simulink model "bolide"  (R2025a)
settings: Solver=VariableStepAuto  StartTime=0.0  StopTime=10.0  RelTol=1e-3
InitFcn:
  | run("init.m")
model workspace (MATLAB code in the model file):
  | % Définition des constantes
  | 
  | rho = 0.04; % rayon des roues
  | k = 0.0854; % constante de couple
  | R = 3.87; % résistance des moteurs
  | d = 0.05; % distance entre le centre des roues et le centre de masse
  | l = 0.16; % distance entre les roues
  | mb = 2; % masse du châssis du robot
  | mw = 0.5; % masse d'une unité
  | M = 2*mw + mb; % masse du robot
  | Ix = 8.48e-3; % moments d'inertie du robot
  | Iz = 1.233e-2;
  | Ixw  = 4.00e-4;    % roue - inertie de rotation autour de l'axe (spin)
  | Izw  = 4.00e-4;    % roue - inertie (même ordre que Ixw)
  | Iyw  = 2.375e-4;   % roue - inertie transversale (axe perpendiculaire au spin)
  | Ipsi = Ix + Iz + Ixw + Izw + mw*(l^2)/2 + Iyw*(l^2)/(2*(rho^2));
  | A = M + 2*Iyw*(rho^2);
  | B = Ipsi + mb*(d^2);
  | D = A*B + 2*(mb*d/2)^2;
settings Model: Creator=arthu  LastModifiedBy=arthu

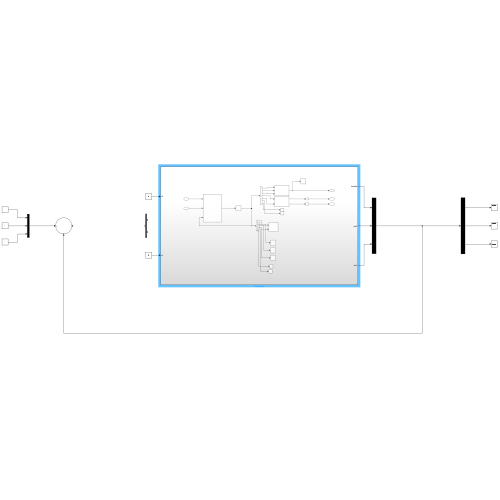
[thumbnail: Simulink's stored preview of the top-level diagram]
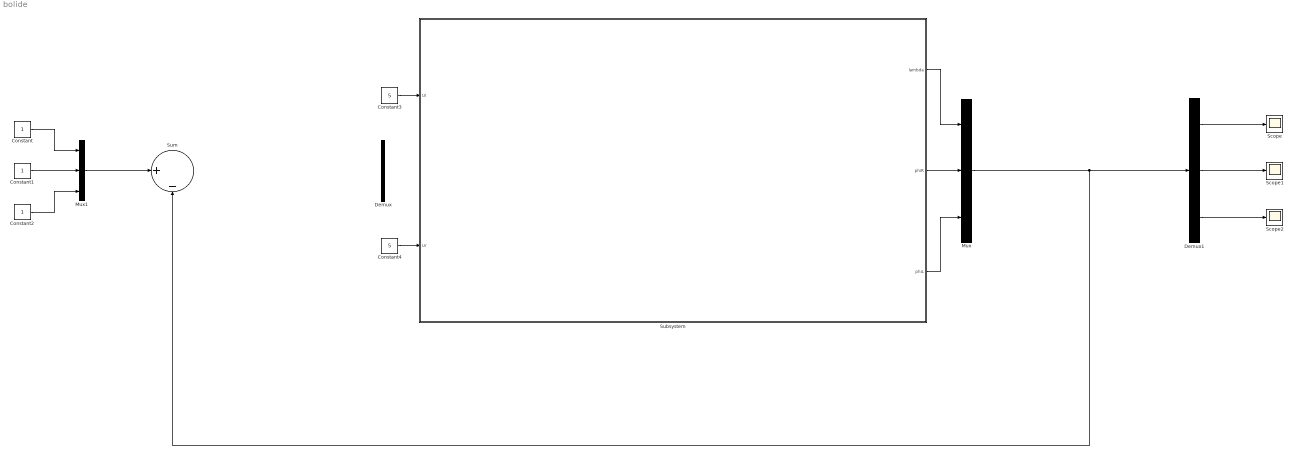
== system bolide ==
  Constant : Constant
  Constant1 : Constant
  Constant2 : Constant
  Constant3 : Constant  Value=5
  Constant4 : Constant  Value=5
  Demux : Demux  Outputs=2
  Demux1 : Demux  Outputs=3
  Mux : Mux  Inputs=3
  Mux1 : Mux  Inputs=3
  Scope : Scope
  Scope1 : Scope
  Scope2 : Scope
      settings: DataLoggingVariableName=ScopeData2
  Subsystem : Subsystem
  Sum : Sum  Inputs=|+-
  wires:
  Subsystem/1(lambda) -> Mux/1
  Subsystem/2(phiR) -> Mux/2
  Subsystem/3(phiL) -> Mux/3
  Mux/1 -> Demux1/1, Sum/2
  Constant/1 -> Mux1/1
  Constant1/1 -> Mux1/2
  Constant2/1 -> Mux1/3
  Mux1/1 -> Sum/1
  Demux1/3 -> Scope2/1
  Demux1/2 -> Scope1/1
  Demux1/1 -> Scope/1
  Constant3/1 -> Subsystem/1(Ul)
  Constant4/1 -> Subsystem/2(Ur)

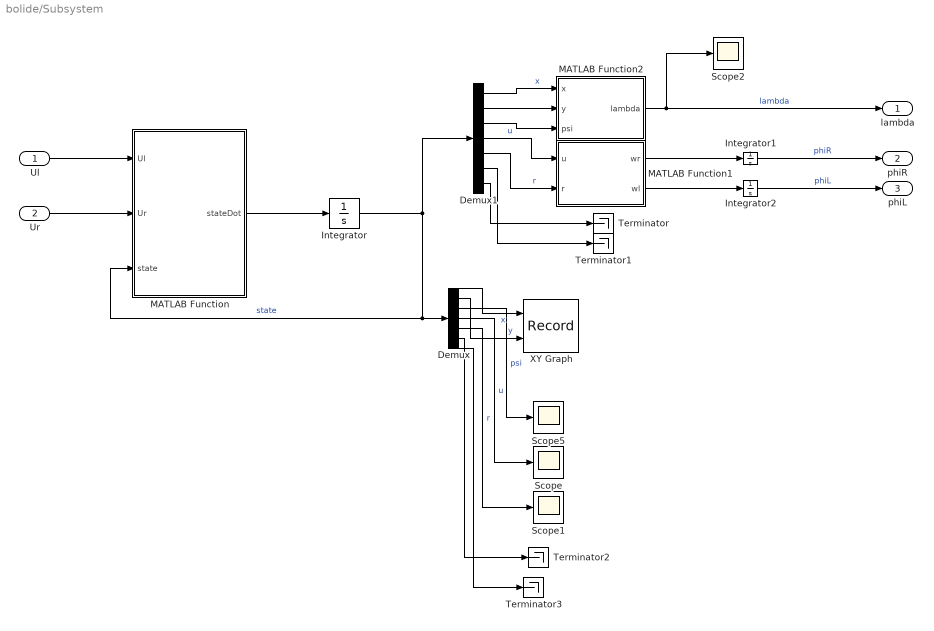
== system bolide/Subsystem ==
  Ul : Inport
  Ur : Inport  Port=2
  Demux : Demux  Outputs=7
  Demux1 : Demux  Outputs=7
  Integrator : Integrator  InitialCondition=[2;0;pi/2;0;0;0;0]
  Integrator1 : Integrator
  Integrator2 : Integrator
  MATLAB Function : MATLAB Function  TreatAsAtomicUnit=on
  MATLAB Function1 : MATLAB Function  TreatAsAtomicUnit=on
  MATLAB Function2 : MATLAB Function  TreatAsAtomicUnit=on
  Scope{,1..2,5} (4 alike) : Scope
      Scope2 settings: ActiveDisplayYMinimum=1.8758001969269686  ActiveDisplayYMaximum=2.2855417469640367  DataLoggingVariableName=ScopeData3
      Scope5 settings: ActiveDisplayYMinimum=-1  ActiveDisplayYMaximum=1  DataLoggingVariableName=ScopeData5
  Terminator{,1..3} (4 alike) : Terminator
  XY Graph : Record  NumPorts=2.0  FileSettingsInternal="{\"entries\":[{\"content\":{\"excelSettings\":{\"content\":{},\"type\":\"Streamout.ExcelSettings\"},\"parquetSettings\":{\"content\":{},\"type\":\"Streamout.ParquetSettings\"}},\"type\":\"Streamout.FileSettingStorage\",\"uuid\":\"\"}],\"packageUris\":[\"http:\\/\\/schema.mathworks.com\\/mf0\\/streamout_blocks\\/R2020a\"],\"version\":\"1.0\"}"  FrameSettings=[0, 0]  Layout=[1 1]  SignalsInternal="{\"entries\":[{\"content\":{\"signals\":[{\"content\":{\"blockPath\":[],\"dimensions\":[1,1],\"domain\":\"\",\"lineColor\":\"#a2142f\",\"plots\":[ 1 ],\"port\":1,\"sid\":[\"\"],\"signalID\":1,\"signalName\":\"x\"},\"type\":\"RecordBlkView.Signal\",\"uuid\":\"\"},{\"content\":{\"blockPath\":[],\"dimensions\":[1,1],\"domain\":\"\",\"lineColor\":\"#139fff\",\"plots\":[ 1 ],\"port\":2,\"sid\":[\"\"],\"signalID\":2,\"signalName\":\"y\"},\"type\":\"RecordBlkView.Signal\",\"uuid\":\"\"}]},\"type\":\"RecordBlkView.InputSignals\",\"uuid\":\"\"}],\"packageUris\":[\"http:\\/\\/schema.mathworks.com\\/mf0\\/streamout_blocks\\/R2020a\"],\"version\":\"1.0\"}"  VisualizationBindings="{\"xyplotplugin\":{\"info\":[{\"series\":[{\"bindingParametersList\":[{\"parameter\":\"X-Axis\",\"signalID\":1,\"signalName\":\"x\"},{\"parameter\":\"Y-Axis\",\"signalID\":2,\"signalName\":\"y\"}],\"seriesID\":0}],\"subplotID\":1}]}}"  CompatibilityTag=XY
  lambda : Outport
  phiR : Outport  Port=2
  phiL : Outport  Port=3
  wires:
  MATLAB Function/1(stateDot) -> Integrator/1
  MATLAB Function1/1(wr) -> Integrator1/1
  Demux1/3 -> MATLAB Function2/3(psi)
  Demux/2 -> XY Graph/2  "y"
  Demux/3 -> Scope5/1  "psi"
  Demux1/1 -> MATLAB Function2/1(x)  "x"
  Demux/4 -> Scope/1  "u"
  MATLAB Function2/1(lambda) -> Scope2/1, lambda/1  "lambda"
  Integrator2/1 -> phiL/1  "phiL"
  Demux/1 -> XY Graph/1  "x"
  Ur/1 -> MATLAB Function/2(Ur)
  Integrator1/1 -> phiR/1  "phiR"
  Integrator/1 -> Demux1/1, Demux/1, MATLAB Function/3(state)  "state"
  Demux1/4 -> MATLAB Function1/1(u)  "u"
  Ul/1 -> MATLAB Function/1(Ul)
  Demux/5 -> Scope1/1  "r"
  Demux1/5 -> MATLAB Function1/2(r)  "r"
  Demux1/2 -> MATLAB Function2/2(y)
  MATLAB Function1/2(wl) -> Integrator2/1
  Demux1/6 -> Terminator1/1
  Demux1/7 -> Terminator/1
  Demux/6 -> Terminator2/1
  Demux/7 -> Terminator3/1

== matlab function bolide/Subsystem/MATLAB Function1 ==
  data: u input; wr output; r input; wl output
function [wr, wl] = fcn(u,r)

% Définition des constantes

rho = 0.04; % rayon des roues
l = 0.16; % distance entre les roues

wr = (2*u + l*r)/(2*rho);
wl = (2*u - l*r)/(2*rho);

== matlab function bolide/Subsystem/MATLAB Function ==
  data: Ul input size=[1 1]; stateDot output size=[7 1]; Ur input size=[1 1]; state input double size=[7 1]
function stateDot = robot(Ul, Ur, state)

% Définition des constantes

rho = 0.04; % rayon des roues
k = 0.0854; % constante de couple
R = 3.87; % résistance des moteurs
d = 0.05; % distance entre le centre des roues et le centre de masse
l = 0.16; % distance entre les roues
L = 0.005;
mb = 2; % masse du châssis du robot
mw = 0.5; % masse d'une unité
M = 2*mw + mb; % masse du robot
Ix = 8.48e-3; % moments d'inertie du robot
Iz = 1.233e-2;
Ixw  = 4.00e-4;    % roue - inertie de rotation autour de l'axe (spin)
Izw  = 4.00e-4;    % roue - inertie (même ordre que Ixw)
Iyw  = 2.375e-4;   % roue - inertie transversale (axe perpendiculaire au spin)
Ipsi = Ix + Iz + Ixw + Izw + mw*(l^2)/2 + Iyw*(l^2)/(2*(rho^2));
A = 1/(M + 2*Iyw*(rho^2));
B = 1/(Ipsi + mb*(d^2));

% Définition des états de notre système

UPlus = Ur + Ul;
UMinus = Ur - Ul;

x = state(1);
y = state(2);
psi = state(3);
u = state(4);
r = state(5);
iPlus = state(6);
iMinus = state(7);

xDot = u * cos(psi);
yDot = u * sin(psi);
psiDot = r;
uDot = -mb*d*(r^2)*A*B +  (A*k/rho)*iPlus;
rDot = (B*l*k/(2*rho))*iMinus + B*mb*d*u*r;
iPlusDot = -(R/L)*iPlus - (2*k*u)/(rho*L) + UPlus/L;
iMinusDot = -(R/L)*iMinus - (k*l*r)/(rho*L) + UMinus/L;

%uDot = (1/A)*((1/rho)*((k/R)*(Ul + Ur) - (2*k^2)/(R*rho)*u) - mb*d*r^2);
%rDot = (1/B)*((l/2*rho)*((k/R)*(Ur - Ul) - (l*k^2)/(R*rho)*r) + mb*d*u*r);
%IdotL = (1/L)*(Ul - R*rho/(2*k)*(A*uDot + mb*d*r^2 - 2/l*(B*rDot - mb*d*u*r)) - k*(2*u - l*r)/(2*rho));
%IdotR = (1/L)*(Ur - R*rho/(2*k)*(A*uDot + mb*d*r^2 + 2/l*(B*rDot - mb*d*u*r)) - k*(2*u + l*r)/(2*rho));

stateDot = [xDot; yDot; psiDot ;uDot ;rDot; iPlusDot; iMinusDot];

== matlab function bolide/Subsystem/MATLAB Function2 ==
  data: x input; lambda output; y input; psi input
function lambda = fcn(x,y,psi)

dCapt = 0.01;

xA = x + dCapt*cos(psi);
yA = y + dCapt*sin(psi);

f_s = @(s) courbe(s, xA, yA, psi);
s0 = 0;
s_sol = fzero(f_s, s0);
disp(s_sol)

g_s = @(z) courbe2(s_sol, xA, yA, psi,z);
z0 = 1;
lambda = fzero(g_s, z0);
